simulink model "granice_nelin_sim"  (R2020a)
settings: Solver=ode5  StartTime=0.0  StopTime=tfin  FixedStep=1e-4  RelTol=1e-3
values from neighbouring files (symbols this model uses):
  F_lower_limit = 0    [FPD_regulacija_nelin_sim_matlab.m]    (also in odredjivanje_granica_varijabli.m; robusni_FPD_regulacija_nelin_sim_matlab.m)
  F_upper_limit = Fe + 1e-3*Fe    (= 3.21211951185)    [FPD_regulacija_nelin_sim_matlab.m]    (also in odredjivanje_granica_varijabli.m = 3.2121089; robusni_FPD_regulacija_nelin_sim_matlab.m)
  K1 = 0.0300    (= 0.03)    [FPD_regulacija_nelin_sim_matlab.m]    (also in odredjivanje_granica_varijabli.m; robusni_FPD_regulacija_nelin_sim_matlab.m)
  K2 = 0.5000    (= 0.5)    [FPD_regulacija_nelin_sim_matlab.m]    (also in odredjivanje_granica_varijabli.m; robusni_FPD_regulacija_nelin_sim_matlab.m)
  mi_max = 1    [FPD_regulacija_nelin_sim_matlab.m]    (also in odredjivanje_granica_varijabli.m; robusni_FPD_regulacija_nelin_sim_matlab.m)
  SF = 10.0000    (= 10)    [FPD_regulacija_nelin_sim_matlab.m]    (also in odredjivanje_granica_varijabli.m; robusni_FPD_regulacija_nelin_sim_matlab.m)
  V = 4.0000    (= 4)    [FPD_regulacija_nelin_sim_matlab.m]    (also in odredjivanje_granica_varijabli.m; robusni_FPD_regulacija_nelin_sim_matlab.m)
  x10 = Xe    (= 4.89066865377)    [FPD_regulacija_nelin_sim_matlab.m]    (also in odredjivanje_granica_varijabli.m = 5; robusni_FPD_regulacija_nelin_sim_matlab.m)
  x20 = Se    (= 0.218662692463)    [FPD_regulacija_nelin_sim_matlab.m]    (also in odredjivanje_granica_varijabli.m = 0; robusni_FPD_regulacija_nelin_sim_matlab.m)
  Y = 0.5000    (= 0.5)    [FPD_regulacija_nelin_sim_matlab.m]    (also in odredjivanje_granica_varijabli.m; robusni_FPD_regulacija_nelin_sim_matlab.m)
undefined symbols (not defined in the file or in its folder): magnitude
settings Model: Creator=anaMceranic  LastModifiedBy=anaMceranic
settings DataIOCC: ReturnWorkspaceOutputs=off

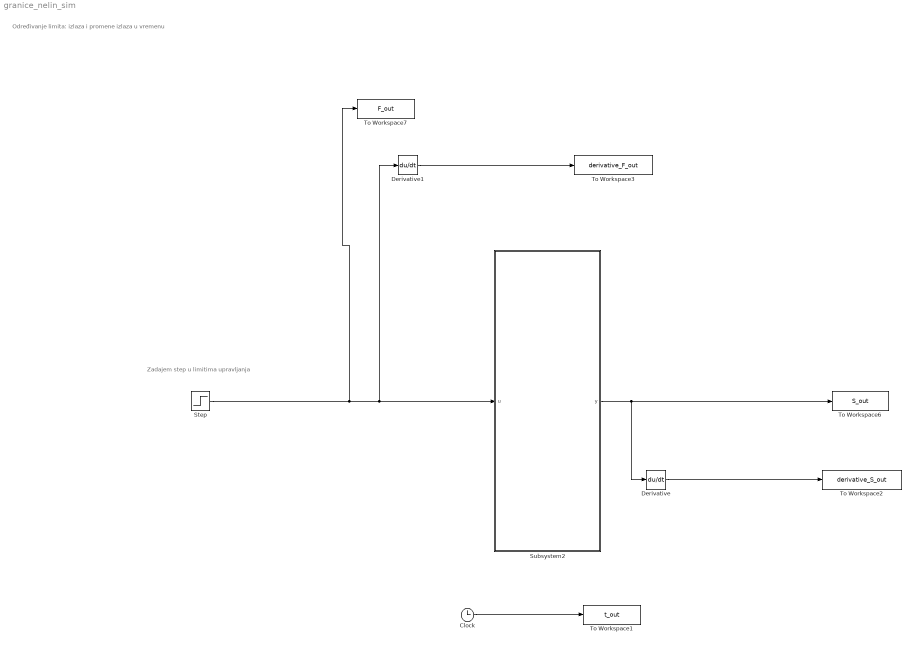
== system granice_nelin_sim ==
  note: Određivanje limita: izlaza i promene izlaza u vremenu
  note: Zadajem step u limitima upravljanja
  Clock : Clock
  Derivative : Derivative
  Derivative1 : Derivative
  Step : Step  Before=F_lower_limit  After=F_upper_limit  SampleTime=0
  Subsystem2 : Subsystem
  To Workspace1 : ToWorkspace  VariableName=t_out  SampleTime=-1
  To Workspace2 : ToWorkspace  VariableName=derivative_S_out  SampleTime=-1
  To Workspace3 : ToWorkspace  VariableName=derivative_F_out  SampleTime=-1
  To Workspace6 : ToWorkspace  VariableName=S_out  SampleTime=-1
  To Workspace7 : ToWorkspace  VariableName=F_out  SampleTime=-1
  wires:
  Clock/1 -> To Workspace1/1
  Step/1 -> Derivative1/1, Subsystem2/1(u), To Workspace7/1
  Subsystem2/1(y) -> To Workspace6/1, Derivative/1
  Derivative/1 -> To Workspace2/1
  Derivative1/1 -> To Workspace3/1

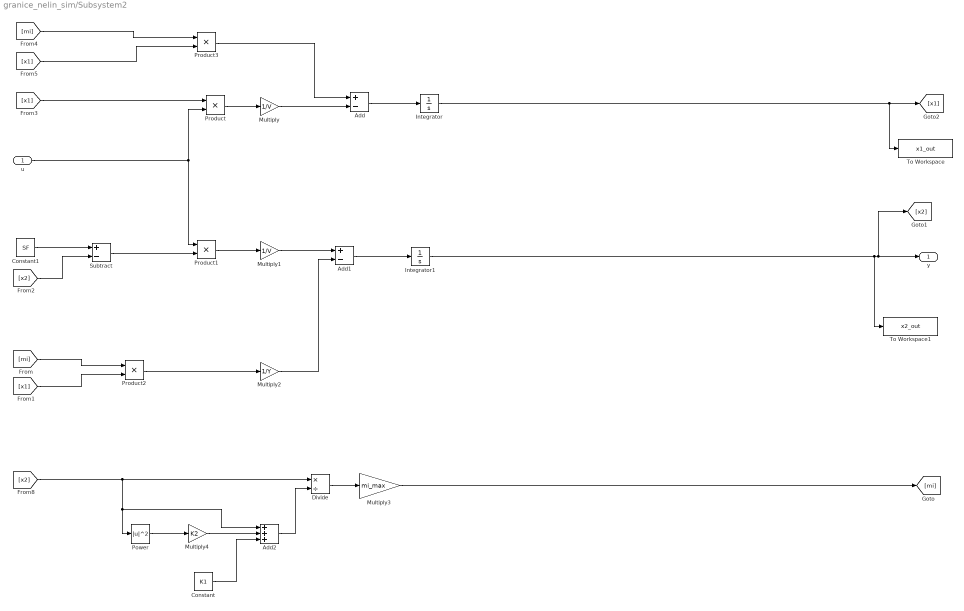
== system granice_nelin_sim/Subsystem2 ==
  u : Inport
  Add : Sum  Inputs=+-
  Add1 : Sum  Inputs=+-
  Add2 : Sum  Inputs=+++
  Constant : Constant  Value=K1
  Constant1 : Constant  Value=SF
  Divide : Product  Inputs=*/
  Integrator : Integrator  InitialCondition=x10
  Integrator1 : Integrator  InitialCondition=x20
  Multiply : Gain  Gain=1/V
  Multiply1 : Gain  Gain=1/V
  Multiply2 : Gain  Gain=1/Y
  Multiply3 : Gain  Gain=mi_max
  Multiply4 : Gain  Gain=K2
  Power : Math  Operator=magnitude^2  SaturateOnIntegerOverflow=on
  Product{,1..3} (4 alike) : Product
  Subtract : Sum  Inputs=+-
  To Workspace : ToWorkspace  VariableName=x1_out  SampleTime=-1
  To Workspace1 : ToWorkspace  VariableName=x2_out  SampleTime=-1
  y : Outport
  wires:
  [x1] -> Product2/2
  Product2/1 -> Multiply2/1
  Multiply/1 -> Add/2
  Add2/1 -> Divide/2
  Constant/1 -> Add2/3
  [x1] -> Product3/2
  Multiply4/1 -> Add2/2
  [mi] -> Product2/1
  Multiply3/1 -> [mi]
  Power/1 -> Multiply4/1
  Constant1/1 -> Subtract/1
  [x2] -> Subtract/2
  Add1/1 -> Integrator1/1
  Multiply2/1 -> Add1/2
  Integrator1/1 -> [x2], y/1, To Workspace1/1
  Divide/1 -> Multiply3/1
  Product3/1 -> Add/1
  u/1 -> Product1/1, Product/2
  [x1] -> Product/1
  Multiply1/1 -> Add1/1
  Product1/1 -> Multiply1/1
  Subtract/1 -> Product1/2
  [x2] -> Divide/1, Add2/1, Power/1
  Add/1 -> Integrator/1
  Product/1 -> Multiply/1
  [mi] -> Product3/1
  Integrator/1 -> To Workspace/1, [x1]
